simulink library "starslibMathOperations"  (R2024b)
settings: Solver=ode45  StartTime=0.0  StopTime=10.0  RelTol=1e-3  EnableMultiTasking=on
libraries: $bdroot x8
(part 1 of 2)
settings Model: Creator=eheim  LastModifiedBy=gryph
settings SolverCC: AlgebraicLoopSolver=TrustRegion
settings DataIOCC: LimitDataPoints=on  SaveFormat=Array  SignalLoggingSaveFormat=ModelDataLogs  ReturnWorkspaceOutputs=off
settings OptimizationCC: ReuseModelBlockBuffer=off  ExpressionDepthLimit=2147483647  LifeSpan=inf
settings DebuggingCC: UnderspecifiedInitializationDetection=Classic  MergeDetectMultiDrivingBlocksExec=none  SolverPrmCheckMsg=warning  FcnCallInpInsideContextMsg=warning  UnconnectedInputMsg=warning  UnconnectedOutputMsg=warning  UnconnectedLineMsg=warning  StateNameClashWarn=warning  SFUnexpectedBacktrackingDiag=warning  SFNoUnconditionalDefaultTransitionDiag=warning  SFExecutionAtInitializationDiag=none  ArithmeticOperatorsInVariantConditions=warning
settings HardwareCC: ProdBitPerPointer=32  ProdBitPerSizeT=32  ProdBitPerPtrDiffT=32  ProdLargestAtomicFloat=None  ProdIntDivRoundTo=Undefined  ProdEndianess=Unspecified  ProdWordSize=32  ProdHWDeviceType=32-bit Generic
settings ModelReferenceCC: PropagateSignalLabelsOutOfModel=off
settings SFSimCC: SimUseLocalCustomCode=off  CustomCodeUndefinedFunction=UseInterfaceOnly
settings RTWCC: RTWUseLocalCustomCode=off  GPUComputeCapability=3.5
settings CodeAppCC: StateflowObjectComments=on
settings GRTTargetCC: TargetLangStandard=C89/C90 (ANSI)  CombineOutputUpdateFcns=off  GRTInterface=on
settings ConfigComp: CovMetricSettings=dw  CovSaveCumulativeToWorkspaceVar=on  CovSaveSingleToWorkspaceVar=on  CovExternalEMLEnable=off  CovSFcnEnable=off

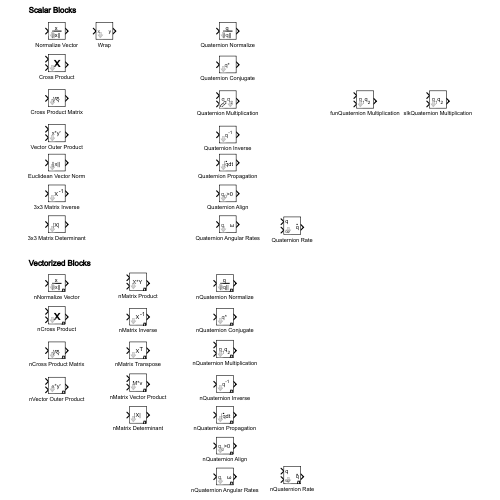
[thumbnail: Simulink's stored preview of the top-level diagram]
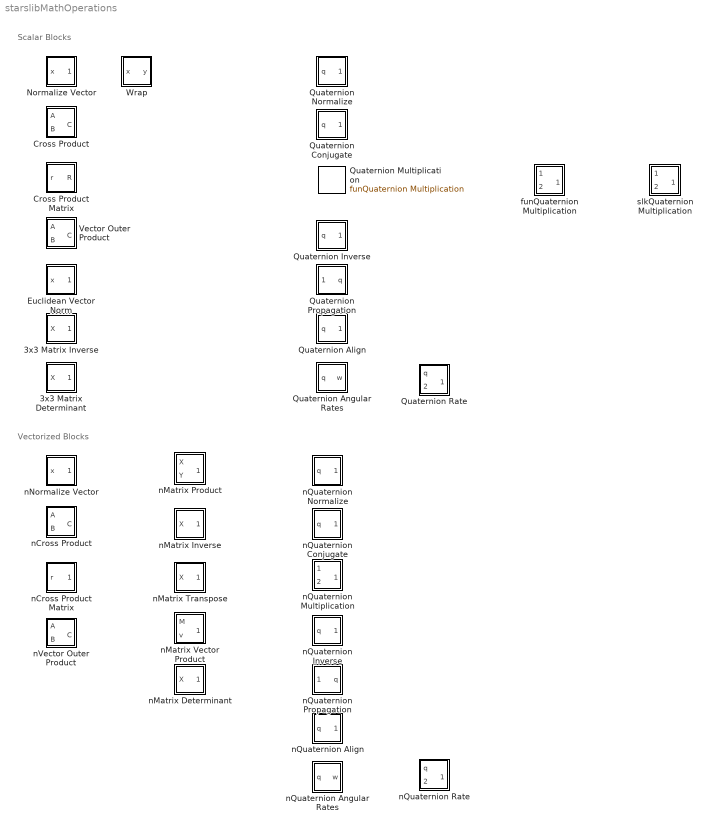
== system starslibMathOperations ==
  note: Scalar Blocks
  note: Vectorized Blocks
  3x3 Matrix Determinant : Subsystem  mask(Matrix Determinant (3x3)){}
      mask help: Determinant of a 3x3 matrix.
      mask Display: text(0.5,0.5,'|X|','HorizontalAlignment','Center','VerticalAlignment','Middle')
  3x3 Matrix Inverse : Subsystem  mask(Matrix Inverse (3x3)){}
      mask help: Inverse of a 3x3 matrix.
      mask Display:
      | text(0.5,0.5,'X','HorizontalAlignment','Center','VerticalAlignment','Middle')
      | text(0.8,0.7,'-1','HorizontalAlignment','Center','VerticalAlignment','Middle')
  Cross Product : Subsystem  mask(Cross Product (1-D)){}
      mask help:
      | Cross product of two 3 element 1-D vectors.  Same as C = cross(A,B) or
      | C = A x B
      |   = [A(2).*B(3) - A(3).*B(2);
      |       A(3).*B(1) - A(1).*B(3);
      |       A(1).*B(2) - A(2).*B(1)];
      mask Display:
      | % plot([0.3 0.7],[0.7 0.3]);
      | % plot([0.3 0.7],[0.3 0.7]);
      |  text(0.575,0.5,'{\fontsize{16}\bfX}','texmode','on','HorizontalAlignment','center',...
      | 	'VerticalAlignment','middle')
  Cross Product Matrix : Subsystem  mask(Cross Product Matrix){n=0}
      mask prompts: n "Hidden variable"
      mask help: Cross product matrix.
      mask Display: text(0.5,0.5,'\{{\itR}\}','texmode', 'on','HorizontalAlignment','Center','VerticalAlignment','Middle')
  Euclidean Vector Norm : Subsystem  mask(Euclidean Norm){dim=1}
      mask prompts: dim "Dimension to take norm"
      mask help: Norm of n-dimensional vector.
      mask Display: text(0.5,0.5,'||x||','texmode', 'on','HorizontalAlignment','Center','VerticalAlignment','Middle')
  Normalize Vector : Subsystem  mask(Normalize Vector){dimnorm=rows, n=1}
      mask prompts: dimnorm "Hidden dimension"; n "Hidden variable"
      mask help: Normalization of 1-dimensional vector.
      mask TypeOptions dimnorm: rows | columns
      mask Display:
      | text(0.5,0.7,'x','HorizontalAlignment','Center','VerticalAlignment','Middle')
      | text(0.5,0.3,'||x||','HorizontalAlignment','Center','VerticalAlignment','Middle')
      | plot([0.2 0.8],[0.5 0.5])
  Quaternion Align : Subsystem  mask(Quaternion Short Path (1-D)){n=0}
      mask prompts: n "Hidden variable"
      mask help: Ensure quaternion transformation takes the shortest possible path. If scalar part is negative the entire quaternion is negated.
      mask Display: text(0.5,0.5,'q_0>0','texmode', 'on','HorizontalAlignment','Center','VerticalAlignment','Middle')
  Quaternion Angular Rates : Subsystem  mask(Quaternion Angular Rates){}
      mask help: Numerically differentiates quaternion and outputs approximation of angular rates.
      mask Display:
      | port_label('input',1,'q','texmode','on')
      | port_label('output',1,'\omega','texmode','on')
  Quaternion Conjugate : Subsystem  mask(Quaternion Conjugate (1-D)){n=0}
      mask prompts: n "Hidden variable"
      mask help: Conjugate of quaternions.
      mask Display: text(0.5,0.5,'q*','HorizontalAlignment','Center','VerticalAlignment','Middle')
  Quaternion Inverse : Subsystem  mask(Quaternion Inverse (1-D)){n=0}
      mask prompts: n "Hidden variable"
      mask help: Inverse of quaternion.
      mask Display: text(0.6,0.6,'q^{-1}','texmode', 'on','HorizontalAlignment','Center','VerticalAlignment','Middle')
  Quaternion Multiplication : $bdroot/funQuaternion Multiplication  n=0
  Quaternion Normalize : Subsystem  mask(Quaternion Normalize (1-D)){n=0}
      mask prompts: n "Hidden variable"
      mask help: Normalization of quaternion.
      mask Display:
      | text(0.5,0.7,'q','HorizontalAlignment','Center','VerticalAlignment','Middle')
      | text(0.5,0.3,'||q||','HorizontalAlignment','Center','VerticalAlignment','Middle')
      | plot([0.2 0.8],[0.5 0.5])
  Quaternion Propagation : Subsystem  mask(Quaternion Propagation (1-D)){qic=[1;0;0;0], k=0.5}
      mask prompts: qic "Initial Quaternion"; k "Stability gain"
      mask help:
      | Integrates dq/dt to propagate a quaternion with algebraic orthonormality stabilization, where:
      |
      |     {dq/dt} = 1/2{q}*{0; omega} + k*lambda*{q}
      |
      | Input, omega is the angular rate of the rotating frame relative to the reference frame in the rotating system's coordinates.
      |
      | Output is the quaternion from the reference coordinate system to the rotating coordinate system.
      |
      | The stability gain parameter, k should be chosen so that k*dT <= 1, where dT is the integration time step.
      mask Help:
      | NASA TN D-5302
      | Zipfel, P. H., Modeling and Simulation of Aerospace Vehicle Dynamics, 2nd Ed., p372
      mask Display:
      | text(0.6,0.5,'\intqdt','texmode', 'on','HorizontalAlignment','Center','VerticalAlignment','Middle')
      | text(0.45,0.85,'\fontsize{20}.','texmode', 'on','HorizontalAlignment','Center','VerticalAlignment','Middle')
  Quaternion Rate : Subsystem  mask(Quaternion Rate){}
      mask help: Computes the quaternion time rate of change.
      mask Display:
      | port_label('input',1,'q')
      | port_label('input',2,'\omega','texmode','on')
      | port_label('output',1,'q')
      | text(0.85,0.80,'\fontsize{20}.','texmode', 'on','HorizontalAlignment','Center','VerticalAlignment','Middle')
  Vector Outer Product : Subsystem  mask(Outer Product (1-D)){n=0}
      mask prompts: n "Hidden variable"
      mask help: Equivilent matlab x(:)*y(:)'
      mask Display: text(0.5,0.5,'x*y''','HorizontalAlignment','Center','VerticalAlignment','Middle')
  Wrap : Subsystem  mask(Wrap Input){R=2*pi, M=0}
      mask prompts: R "Range of output"; M "Minimum of output"
      mask help: Wraps input to specified range with specified minimum.
  funQuaternion Multiplication : Subsystem  mask(Quaternion Multiplication (1-D)){n=0}
      mask prompts: n "Hidden variable"
      mask help: Quaternion multiplication.
      mask Display: text(0.5,0.5,'q_1q_2','texmode','on','HorizontalAlignment','Center','VerticalAlignment','Middle')
  nCross Product : Subsystem  mask(nCross Product){n=1}
      mask prompts: n "Number of Vectors"
      mask help:
      | Cross product of each respective column for two 3xN matricies.  Same as C = cross(A,B) or
      | C = A x B
      |   = [A(2,:).*B(3,:) - A(3,:).*B(2,:);
      |       A(3,:).*B(1,:) - A(1,:).*B(3,:);
      |       A(1,:).*B(2,:) - A(2,:).*B(1,:)];
      mask Display:
      | % plot([0.3 0.7],[0.7 0.3]);
      | % plot([0.3 0.7],[0.3 0.7]);
      | text(0.575,0.5,'{\fontsize{16}\bfX}','texmode','on','HorizontalAlignment','center','VerticalAlignment','middle')
      | text(1,0,'\bf\it{n}','texmode','on','HorizontalAlignment','Right','VerticalAlignment','base')
  nCross Product Matrix : Subsystem  mask(nCross Product Matrix){n=1}
      mask prompts: n "Number of Vectors"
      mask help: Each column corresponds is the cross product matrix, R reshaped into a vector by columns, i.e. R(:). Inputs must be 3xN in size. Outputs are 9xN in size.
      mask init:
      | A = diag([0 1 -1 -1 0 1 1 -1 0]);
      mask Display:
      | text(0.5,0.5,'\{{\itR}\}','texmode', 'on','HorizontalAlignment','Center','VerticalAlignment','Middle')
      | text(1,0,'\bf\it{n}','texmode','on','HorizontalAlignment','Right','VerticalAlignment','base')
  nMatrix Determinant : Subsystem  mask(nMatrix Determinant){n=1}
      mask prompts: n "Number of Matricies"
      mask help: Determinant of set of matricies.
      mask Display:
      | text(0.5,0.5,'|X|','HorizontalAlignment','Center','VerticalAlignment','Middle')
      | text(1,0,'\bf\it{n}','texmode','on','HorizontalAlignment','Right','VerticalAlignment','base')
  nMatrix Inverse : Subsystem  mask(nMatrix Product){n=1}
      mask prompts: n "Number of Matricies"
      mask help:
      | Output reshape(XY(:,k),3,3)
      | corresponds to the matrix product
      | reshape(X(:,k),3,3)*reshape(Y(:,k),3,3)
      |
      | Note: This block has no divide by zero protection.
      mask Display:
      | text(0.5,0.5,'X','HorizontalAlignment','Center','VerticalAlignment','Middle')
      | text(0.8,0.7,'-1','HorizontalAlignment','Center','VerticalAlignment','Middle')
      | text(1,0,'\bf\it{n}','texmode','on','HorizontalAlignment','Right','VerticalAlignment','base')
  nMatrix Product : Subsystem  mask(nMatrix Product){n=1}
      mask prompts: n "Number of Matricies"
      mask help:
      | Output reshape(XY(:,k),3,3)
      | corresponds to the matrix product
      | reshape(X(:,k),3,3)*reshape(Y(:,k),3,3)
      mask Display:
      | text(0.5,0.5,'X*Y','HorizontalAlignment','Center','VerticalAlignment','Middle')
      | text(1,0,'\bf\it{n}','texmode','on','HorizontalAlignment','Right','VerticalAlignment','base')
  nMatrix Transpose : Subsystem  mask(nMatrix Transpose){n=1}
      mask prompts: n "Number of Matricies"
      mask help:
      | Output reshape(AT(:,k),3,3) corresponds
      | to the transpose of reshape(A(:,k),3,3).
      mask Display:
      | text(0.5,0.5,'X','HorizontalAlignment','Center','VerticalAlignment','Middle')
      | text(0.75,0.65,'T','HorizontalAlignment','Center','VerticalAlignment','Middle')
      | text(1,0,'\bf\it{n}','texmode','on','HorizontalAlignment','Right','VerticalAlignment','base')
  nMatrix Vector Product : Subsystem  mask(nMatrix Vector Product){n=1}
      mask prompts: n "Number of Matricies"
      mask help:
      | Output AV(:,k) corresponds to
      | the matrix-vector product
      | reshape(A(:,k),3,3)*V(:,k)
      mask Display:
      | text(0.5,0.5,'M*v','HorizontalAlignment','Center','VerticalAlignment','Middle')
      | text(1,0,'\bf\it{n}','texmode','on','HorizontalAlignment','Right','VerticalAlignment','base')
  nNormalize Vector : Subsystem  mask(nNormalize Vector){dimnorm=rows, n=[3, 1]}
      mask prompts: dimnorm "Dimension to normalize"; n "Dimensions of input [m n]"
      mask help: Normalization of either rows or columns of a 2-dimensional matrix.
      mask init:
      | % Repleat magnitude array, M by A*M*B
      | switch dimnorm
      |     case 1
      |         A = ones(n(1),1);
      |         B = eye(n(2));
      |     case 2
      |         A = eye(n(1));
      |         B  = ones(1,n(2));
      | end
      mask TypeOptions dimnorm: rows | columns
      mask Display:
      | text(0.5,0.7,'x','HorizontalAlignment','Center','VerticalAlignment','Middle')
      | text(0.5,0.3,'||x||','HorizontalAlignment','Center','VerticalAlignment','Middle')
      | plot([0.2 0.8],[0.5 0.5])
      | text(1,0,'\bf\it{n}','texmode','on','HorizontalAlignment','Right','VerticalAlignment','base')
  nQuaternion Align : Subsystem  mask(nQuaternion Align){n=1}
      mask prompts: n "Number of Quaternions"
      mask help: Ensure quaternion transformation takes the shortest possible path. If scalar part is negative the entire quaternion is negated.
      mask Display:
      | text(0.5,0.5,'q_0>0','texmode', 'on','HorizontalAlignment','Center','VerticalAlignment','Middle')
      | text(1,0,'\bf\it{n}','texmode','on','HorizontalAlignment','Right','VerticalAlignment','base')
  nQuaternion Angular Rates : Subsystem  mask(nQuaternion Angular Rates){n=0}
      mask prompts: n "Number of Quaternions"
      mask help: Numerically differentiates quaternion and outputs approximation of angular rates.
      mask Display:
      | text(1,0,'\bf\it{n}','texmode','on','HorizontalAlignment','Right','VerticalAlignment','base')
      | port_label('input',1,'q','texmode','on')
      | port_label('output',1,'\omega','texmode','on')
  nQuaternion Conjugate : Subsystem  mask(nQuaternion Conjugate){n=1}
      mask prompts: n "Number of Quaternions"
      mask help: Conjugate of quaternions.
      mask Display:
      | text(0.5,0.5,'q*','HorizontalAlignment','Center','VerticalAlignment','Middle')
      | text(1,0,'\bf\it{n}','texmode','on','HorizontalAlignment','Right','VerticalAlignment','base')
  nQuaternion Inverse : Subsystem  mask(nQuaternion Inverse){n=1}
      mask prompts: n "Number of Quaternions"
      mask help: Inverse of quaternions.
      mask Display:
      | text(0.6,0.6,'q^{-1}','texmode', 'on','HorizontalAlignment','Center','VerticalAlignment','Middle')
      | text(1,0,'\bf\it{n}','texmode','on','HorizontalAlignment','Right','VerticalAlignment','base')
  nQuaternion Multiplication : Subsystem  mask(nQuaternion Multiplication){n=1}
      mask prompts: n "Number of Quaternions"
      mask help:
      | Quaternion multiplication of two sets of quaternions
      | inputted by 2 (4 x nQuat) matrices
      mask Display:
      | text(0.5,0.5,'q_1q_2','texmode','on','HorizontalAlignment','Center','VerticalAlignment','Middle')
      | text(1,0,'\bf\it{n}','texmode','on','HorizontalAlignment','Right','VerticalAlignment','base')
  nQuaternion Normalize : Subsystem  mask(nQuaternion Normalize){n=1}
      mask prompts: n "Number of Quaternions"
      mask help: Normalization of quaternion.
      mask Display:
      | text(0.5,0.7,'q','HorizontalAlignment','Center','VerticalAlignment','Middle')
      | text(0.5,0.3,'||q||','HorizontalAlignment','Center','VerticalAlignment','Middle')
      | plot([0.2 0.8],[0.5 0.5])
      | text(1,0,'\bf\it{n}','texmode','on','HorizontalAlignment','Right','VerticalAlignment','base')
  nQuaternion Propagation : Subsystem  mask(nQuaternion Propagation){n=1, q0=[1;0;0;0], k=0.5}
      mask prompts: n "Number of Quaternions"; q0 "Initial Quaternion(s)"; k "Stability gain"
      mask help:
      | Integrates dq/dt to propagate a quaternion with algebraic orthonormality stabilization, where:
      |
      |     {dq/dt} = 1/2{q}*{0; omega} + k*lambda*{q}
      |
      | Input, omega is the angular rate of the rotating frame relative to the reference frame in the rotating system's coordinates.
      |
      | Output is the quaternion from the reference coordinate system to the rotating coordinate system.
      |
      | The stability gain parameter, k should be chosen so that k*dT <= 1, where dT is the integration time step.
      mask Help:
      | NASA TN D-5302
      | Zipfel, P. H., Modeling and Simulation of Aerospace Vehicle Dynamics, 2nd Ed., p372
      mask Display:
      | text(0.6,0.5,'\intqdt','texmode', 'on','HorizontalAlignment','Center','VerticalAlignment','Middle')
      | text(0.45,0.85,'\fontsize{20}.','texmode', 'on','HorizontalAlignment','Center','VerticalAlignment','Middle')
      | text(1,0,'\bf\it{n}','texmode','on','HorizontalAlignment','Right','VerticalAlignment','base')
  nQuaternion Rate : Subsystem  mask(Quaternion Rate){n=1}
      mask prompts: n "Number of quaternions in input"
      mask help: Computes the quaternion time rate of change.
      mask Display:
      | port_label('input',1,'q')
      | port_label('input',2,'\omega','texmode','on')
      | port_label('output',1,'q')
      | text(0.85,0.80,'\fontsize{20}.','texmode', 'on','HorizontalAlignment','Center','VerticalAlignment','Middle')
      | text(1,0,'\bf\it{n}','texmode','on','HorizontalAlignment','Right','VerticalAlignment','base')
  nVector Outer Product : Subsystem  mask(nOuter Product){n=1}
      mask prompts: n "Number of Vectors"
      mask help:
      | reshape(OP(:,k),3,3) corresponds
      | to the outer product matrix defined
      | by input X(:,k)*Y(:,k)'.
      mask Display:
      | text(0.5,0.5,'x*y''','HorizontalAlignment','Center','VerticalAlignment','Middle')
      | text(1,0,'\bf\it{n}','texmode','on','HorizontalAlignment','Right','VerticalAlignment','base')
  slkQuaternion Multiplication : Subsystem  mask(Quaternion Multiplication (1-D)){n=0}
      mask prompts: n "Hidden variable"
      mask help: Quaternion multiplication.
      mask Display: text(0.5,0.5,'q_1q_2','texmode','on','HorizontalAlignment','Center','VerticalAlignment','Middle')

== system starslibMathOperations/3x3 Matrix Determinant ==
  X : Inport  PortDimensions=[3,3]
  Reshape : Reshape  OutputDimensionality=Column vector (2-D)
  nMatrix Determinant : $bdroot/nMatrix Determinant  n=1
  inv(X) : Outport  PortDimensions=[1,1]
  wires:
  Reshape/1 -> nMatrix Determinant/1
  X/1 -> Reshape/1
  nMatrix Determinant/1 -> inv(X)/1

== system starslibMathOperations/3x3 Matrix Inverse ==
  X : Inport
  3x3 Matrix Determinant : $bdroot/3x3 Matrix Determinant
  Assertion : Assertion  AssertionFailFcn="disp('Matrix inverse failed.  Matrix is singular.')"
  Product : Product  Inputs=/  Multiplication=Matrix(*)  RndMeth=Zero
  inv(X) : Outport
  wires:
  Product/1 -> inv(X)/1
  X/1 -> Product/1, 3x3 Matrix Determinant/1
  3x3 Matrix Determinant/1 -> Assertion/1

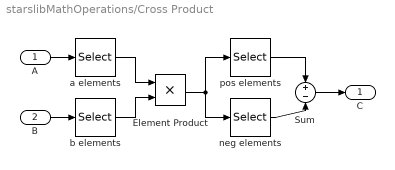
== system starslibMathOperations/Cross Product ==
  A : Inport
  B : Inport  Port=2
  Element Product : Product  RndMeth=Zero
  Sum : Sum  Inputs=+|-
  a elements : Selector  InputPortWidth=3  IndexOptions=Index vector (dialog)  Indices=[2 3 1 3 1 2]  OutputSizes=1
  b elements : Selector  InputPortWidth=3  IndexOptions=Index vector (dialog)  Indices=[3 1 2 2 3 1]  OutputSizes=1
  neg elements : Selector  InputPortWidth=6  IndexOptions=Index vector (dialog)  Indices=[4:6]  OutputSizes=1
  pos elements : Selector  InputPortWidth=6  IndexOptions=Index vector (dialog)  Indices=[1:3]  OutputSizes=1
  C : Outport
  wires:
  a elements/1 -> Element Product/1
  b elements/1 -> Element Product/2
  Element Product/1 -> pos elements/1, neg elements/1
  pos elements/1 -> Sum/1
  neg elements/1 -> Sum/2
  Sum/1 -> C/1
  A/1 -> a elements/1
  B/1 -> b elements/1

== system starslibMathOperations/Cross Product Matrix ==
  r : Inport
  Constant : Constant  Value=[0 1 -1 -1 0 1 1 -1 0]
  Product : Product  RndMeth=Zero
  Reshape : Reshape  OutputDimensionality=Customize  OutputDimensions=[3,3]
  Selector : Selector  InputPortWidth=3  IndexOptions=Index vector (dialog)  Indices=[1 3 2 3 2 1 2 1 3]  OutputSizes=1
  R : Outport  PortDimensions=[3,3]
  wires:
  Reshape/1 -> R/1
  Product/1 -> Reshape/1
  Selector/1 -> Product/2
  r/1 -> Selector/1
  Constant/1 -> Product/1

== system starslibMathOperations/Euclidean Vector Norm ==
  x : Inport
  Math Function : Math  Operator=square  SignedPower=on
  Sqrt : Sqrt
  Sum of Elements : Sum  Inputs=+  CollapseMode=Specified dimension  CollapseDim=dim
  ||x|| : Outport
  wires:
  Sqrt/1 -> ||x||/1
  x/1 -> Math Function/1
  Sum of Elements/1 -> Sqrt/1
  Math Function/1 -> Sum of Elements/1

== system starslibMathOperations/Normalize Vector ==
  x : Inport
  Divide : Product  Inputs=*/
  Math Function : Math  Operator=square  SignedPower=on
  Sqrt : Sqrt
  Sum of Elements : Sum  Inputs=+  CollapseDim=dim
  ux : Outport
  wires:
  Sum of Elements/1 -> Sqrt/1
  Math Function/1 -> Sum of Elements/1
  x/1 -> Math Function/1, Divide/1
  Divide/1 -> ux/1
  Sqrt/1 -> Divide/2

== system starslibMathOperations/Quaternion Align ==
  q : Inport
  Selector2 : Selector  InputPortWidth=4  IndexOptions=Index vector (dialog)  Indices=1  OutputSizes=1
  Switch : Switch  Criteria=u2 > Threshold  ZeroCross=off  SaturateOnIntegerOverflow=off  InputSameDT=off
  Unary Minus : UnaryMinus
  short(q) : Outport
  wires:
  Unary Minus/1 -> Switch/3
  Selector2/1 -> Switch/2
  Switch/1 -> short(q)/1
  q/1 -> Unary Minus/1, Switch/1, Selector2/1

== system starslibMathOperations/Quaternion Angular Rates ==
  q : Inport  PortDimensions=4
  Derivative1 : Derivative
  Gain : Gain  Gain=2
  Gain1 : Gain  Gain=[-1 -1 -1, 1 -1 1, 1 1 -1, -1 1 1]'
  Product3 : Product  Multiplication=Matrix(*)  RndMeth=Zero
  Reshape : Reshape  OutputDimensionality=Customize  OutputDimensions=[3,4]
  Selector3 : Selector  InputPortWidth=4  IndexOptions=Index vector (dialog)  Indices=[2 3 4, 1 4 3, 4 1 2, 3 2 1]  OutputSizes=1
  w : Outport  PortDimensions=3
  wires:
  Selector3/1 -> Gain1/1
  Gain1/1 -> Reshape/1
  Reshape/1 -> Product3/1
  q/1 -> Selector3/1, Derivative1/1
  Product3/1 -> Gain/1
  Gain/1 -> w/1
  Derivative1/1 -> Product3/2

== system starslibMathOperations/Quaternion Conjugate ==
  q : Inport
  Constant : Constant  Value=[1 -1 -1 -1]
  Product : Product  RndMeth=Zero
  q* : Outport
  wires:
  Product/1 -> q*/1
  Constant/1 -> Product/1
  q/1 -> Product/2

== system starslibMathOperations/Quaternion Inverse ==
  q : Inport
  Math Function1 : Math  Operator=square  SignedPower=on
  Product : Product  Inputs=*/  RndMeth=Zero
  Quaternion Conjugate : $bdroot/Quaternion Conjugate  n=0
  Sum of Elements : Sum  Inputs=+
  inv(q) : Outport
  wires:
  Math Function1/1 -> Sum of Elements/1
  Quaternion Conjugate/1 -> Product/1
  q/1 -> Math Function1/1, Quaternion Conjugate/1
  Sum of Elements/1 -> Product/2
  Product/1 -> inv(q)/1

== system starslibMathOperations/Quaternion Normalize ==
  q : Inport
  Math Function1 : Math  Operator=square  SignedPower=on
  Product : Product  Inputs=*/  RndMeth=Zero
  Sqrt : Sqrt
  Sum of Elements : Sum  Inputs=+
  q/||q|| : Outport
  wires:
  Math Function1/1 -> Sum of Elements/1
  Sum of Elements/1 -> Sqrt/1
  Product/1 -> q/||q||/1
  Sqrt/1 -> Product/2
  q/1 -> Math Function1/1, Product/1

== system starslibMathOperations/Quaternion Propagation ==
  Omega : Inport
  Integrator : Integrator  InitialCondition=qic
  Orthonormality Error : Subsystem
      mask Display: text(0.5,0.5,'\lambda','texmode', 'on','HorizontalAlignment','Center','VerticalAlignment','Middle')
  Product : Product  RndMeth=Zero
  Quaternion Rate : $bdroot/Quaternion Rate
  Sum : Sum  Inputs=|++
  k : Gain  Gain=k
  q : Outport
  wires:
  Product/1 -> Sum/2
  k/1 -> Product/1
  Orthonormality Error/1(lambda) -> k/1
  Quaternion Rate/1 -> Sum/1
  Sum/1 -> Integrator/1
  Integrator/1 -> Product/2, Quaternion Rate/1, Orthonormality Error/1(q), q/1
  Omega/1 -> Quaternion Rate/2

== system starslibMathOperations/Quaternion Rate ==
  q : Inport
  Omega : Inport  Port=2
  Gain : Gain  Gain=0.5
  Subsystem6 : Subsystem  mask(Quat Mult for two special sets of quaternions){}
      mask help:
      | Quaternion multiplication of two sets of quaternions. First element assumed
      | zero of second Quaternion.  Input only last three elements
      | of second quaternion.
      mask Display:
      | disp('Quat Mult\n q0=0')
      | port_label('input',1,'p')
      | port_label('input',2,'q')
      | port_label('output',1,'p*q')
  qdt : Outport
  wires:
  Omega/1 -> Subsystem6/2(q)
  Gain/1 -> qdt/1
  q/1 -> Subsystem6/1(p)
  Subsystem6/1(p * q) -> Gain/1

== system starslibMathOperations/Vector Outer Product ==
  A : Inport
  B : Inport  Port=2
  Element Product : Product  RndMeth=Zero
  Reshape : Reshape  OutputDimensionality=Customize  OutputDimensions=[3,3]
  a elements : Selector  InputPortWidth=3  IndexOptions=Index vector (dialog)  Indices=[1 2 3 1 2 3 1 2 3]  OutputSizes=1
  b elements : Selector  InputPortWidth=3  IndexOptions=Index vector (dialog)  Indices=[1 1 1 2 2 2 3 3 3]  OutputSizes=1
  C : Outport
  wires:
  Reshape/1 -> C/1
  a elements/1 -> Element Product/1
  b elements/1 -> Element Product/2
  A/1 -> a elements/1
  B/1 -> b elements/1
  Element Product/1 -> Reshape/1

== system starslibMathOperations/Wrap ==
  x : Inport
  Min : Constant  Value=M  VectorParams1D=off
  Range : Constant  Value=R  VectorParams1D=off
  Sum : Sum  Inputs=|+-
  Sum1 : Sum  Inputs=|++
  mod : Math  Operator=mod  SignedPower=on
  y : Outport
  wires:
  Sum1/1 -> y/1
  x/1 -> Sum/1
  Sum/1 -> mod/1
  Range/1 -> mod/2
  mod/1 -> Sum1/1
  Min/1 -> Sum1/2, Sum/2

== system starslibMathOperations/funQuaternion Multiplication ==
  q1 : Inport
  q2 : Inport  Port=2
  Quaternion Multiplication : MATLAB Function  TreatAsAtomicUnit=on
  q1q2 : Outport
  wires:
  Quaternion Multiplication/1(q1q2) -> q1q2/1
  q2/1 -> Quaternion Multiplication/2(q2)
  q1/1 -> Quaternion Multiplication/1(q1)

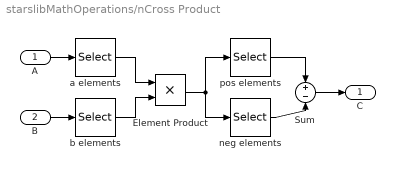
== system starslibMathOperations/nCross Product ==
  A : Inport  PortDimensions=[3,n]
  B : Inport  Port=2  PortDimensions=[3,n]
  Element Product : Product  RndMeth=Zero
  Sum : Sum  Inputs=+|-
  a elements : Selector  NumberOfDimensions=2  InputPortWidth=3  IndexOptions=Index vector (dialog),Select all  Indices=[2 3 1 3 1 2],1  OutputSizes=1,1
  b elements : Selector  NumberOfDimensions=2  InputPortWidth=3  IndexOptions=Index vector (dialog),Select all  Indices=[3 1 2 2 3 1],1  OutputSizes=1,1
  neg elements : Selector  NumberOfDimensions=2  InputPortWidth=3  IndexOptions=Index vector (dialog),Select all  Indices=[4:6],1  OutputSizes=1,1
  pos elements : Selector  NumberOfDimensions=2  InputPortWidth=3  IndexOptions=Index vector (dialog),Select all  Indices=[1:3],1  OutputSizes=1,1
  C : Outport  PortDimensions=[3,n]
  wires:
  a elements/1 -> Element Product/1
  b elements/1 -> Element Product/2
  Element Product/1 -> pos elements/1, neg elements/1
  pos elements/1 -> Sum/1
  neg elements/1 -> Sum/2
  Sum/1 -> C/1
  A/1 -> a elements/1
  B/1 -> b elements/1

== system starslibMathOperations/nCross Product Matrix ==
  r : Inport  PortDimensions=[3,n]
  Constant : Constant  Value=A
  Product : Product  Multiplication=Matrix(*)  RndMeth=Zero
  Selector : Selector  NumberOfDimensions=2  InputPortWidth=3  IndexOptions=Index vector (dialog),Select all  Indices=[1 3 2 3 2 1 2 1 3],1  OutputSizes=1,1
  nR(:) : Outport  PortDimensions=[9,n]
  wires:
  Product/1 -> nR(:)/1
  Selector/1 -> Product/2
  r/1 -> Selector/1
  Constant/1 -> Product/1

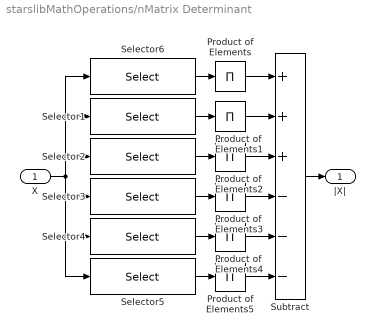
== system starslibMathOperations/nMatrix Determinant ==
  X : Inport  PortDimensions=[9,n]
  Product of Elements{,1..5} (6 alike) : Product  Inputs=*  CollapseMode=Specified dimension
  Selector1 : Selector  NumberOfDimensions=2  InputPortWidth=3  IndexOptions=Index vector (dialog),Select all  Indices=[4 8 3],1  OutputSizes=1,1
  Selector2 : Selector  NumberOfDimensions=2  InputPortWidth=3  IndexOptions=Index vector (dialog),Select all  Indices=[7 2 6],1  OutputSizes=1,1
  Selector3 : Selector  NumberOfDimensions=2  InputPortWidth=3  IndexOptions=Index vector (dialog),Select all  Indices=[7 5 3],1  OutputSizes=1,1
  Selector4 : Selector  NumberOfDimensions=2  InputPortWidth=3  IndexOptions=Index vector (dialog),Select all  Indices=[4 2 9],1  OutputSizes=1,1
  Selector5 : Selector  NumberOfDimensions=2  InputPortWidth=3  IndexOptions=Index vector (dialog),Select all  Indices=[1 8 6],1  OutputSizes=1,1
  Selector6 : Selector  NumberOfDimensions=2  InputPortWidth=3  IndexOptions=Index vector (dialog),Select all  Indices=[1 5 9],1  OutputSizes=1,1
  Subtract : Sum  Inputs=+++---
  |X| : Outport  PortDimensions=[1,n]
  wires:
  Selector6/1 -> Product of Elements/1
  Selector1/1 -> Product of Elements1/1
  Selector2/1 -> Product of Elements2/1
  Selector3/1 -> Product of Elements3/1
  Selector4/1 -> Product of Elements4/1
  Selector5/1 -> Product of Elements5/1
  X/1 -> Selector2/1, Selector6/1, Selector1/1, Selector3/1, Selector5/1, Selector4/1
  Product of Elements/1 -> Subtract/1
  Product of Elements1/1 -> Subtract/2
  Product of Elements2/1 -> Subtract/3
  Product of Elements3/1 -> Subtract/4
  Product of Elements4/1 -> Subtract/5
  Product of Elements5/1 -> Subtract/6
  Subtract/1 -> |X|/1

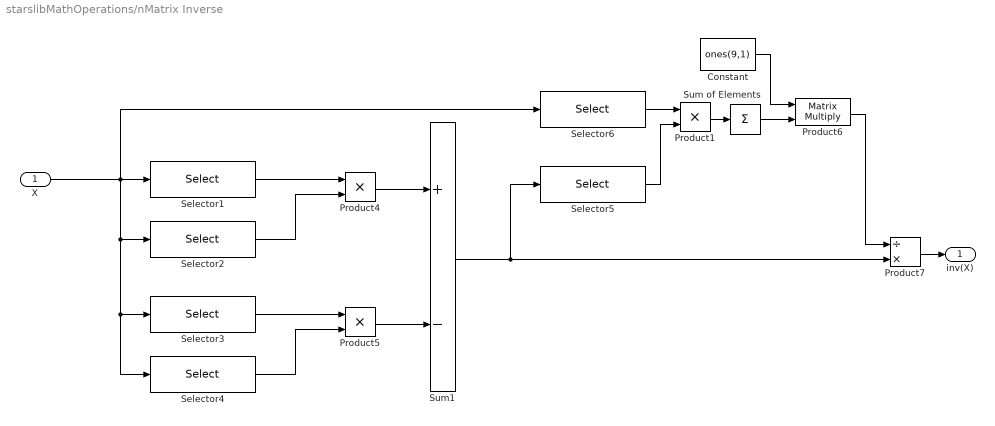
== system starslibMathOperations/nMatrix Inverse ==
  X : Inport  PortDimensions=[9,n]
  Constant : Constant  Value=ones(9,1)  VectorParams1D=off
  Product1 : Product  RndMeth=Zero
  Product4 : Product  RndMeth=Zero
  Product5 : Product  RndMeth=Zero
  Product6 : Product  Multiplication=Matrix(*)  RndMeth=Zero
  Product7 : Product  Inputs=/*  RndMeth=Zero
  Selector1 : Selector  NumberOfDimensions=2  InputPortWidth=3  IndexOptions=Index vector (dialog),Select all  Indices=[5 8 2 7 1 4 4 7 1],1  OutputSizes=1,1
  Selector2 : Selector  NumberOfDimensions=2  InputPortWidth=3  IndexOptions=Index vector (dialog),Select all  Indices=[9 3 6 6 9 3 8 2 5],1  OutputSizes=1,1
  Selector3 : Selector  NumberOfDimensions=2  InputPortWidth=3  IndexOptions=Index vector (dialog),Select all  Indices=[8 2 5 4 7 1 7 1 4],1  OutputSizes=1,1
  Selector4 : Selector  NumberOfDimensions=2  InputPortWidth=3  IndexOptions=Index vector (dialog),Select all  Indices=[6 9 3 9 3 6 5 8 2],1  OutputSizes=1,1
  Selector5 : Selector  NumberOfDimensions=2  InputPortWidth=3  IndexOptions=Index vector (dialog),Select all  Indices=[1 2 3],1  OutputSizes=1,1
  Selector6 : Selector  NumberOfDimensions=2  InputPortWidth=3  IndexOptions=Index vector (dialog),Select all  Indices=[1 4 7],1  OutputSizes=1,1
  Sum of Elements : Sum  Inputs=+  CollapseMode=Specified dimension
  Sum1 : Sum  Inputs=+-
  inv(X) : Outport  PortDimensions=[9,n]
  wires:
  Product7/1 -> inv(X)/1
  Product6/1 -> Product7/1
  Constant/1 -> Product6/1
  Sum of Elements/1 -> Product6/2
  Product1/1 -> Sum of Elements/1
  Selector5/1 -> Product1/2
  Selector6/1 -> Product1/1
  Sum1/1 -> Product7/2, Selector5/1
  Product5/1 -> Sum1/2
  Product4/1 -> Sum1/1
  Selector4/1 -> Product5/2
  Selector3/1 -> Product5/1
  Selector2/1 -> Product4/2
  Selector1/1 -> Product4/1
  X/1 -> Selector6/1, Selector2/1, Selector4/1, Selector3/1, Selector1/1

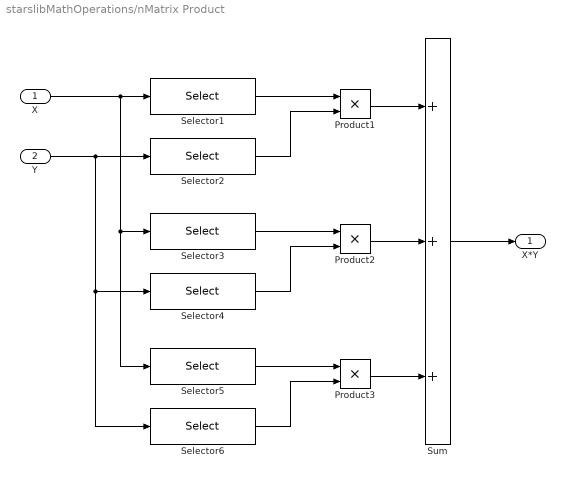
== system starslibMathOperations/nMatrix Product ==
  X : Inport  PortDimensions=[9,n]
  Y : Inport  Port=2  PortDimensions=[9,n]
  Product1 : Product  RndMeth=Zero
  Product2 : Product  RndMeth=Zero
  Product3 : Product  RndMeth=Zero
  Selector1 : Selector  NumberOfDimensions=2  InputPortWidth=3  IndexOptions=Index vector (dialog),Select all  Indices=[1 2 3 1 2 3 1 2 3],1  OutputSizes=1,1
  Selector2 : Selector  NumberOfDimensions=2  InputPortWidth=3  IndexOptions=Index vector (dialog),Select all  Indices=[1 1 1 4 4 4 7 7 7],1  OutputSizes=1,1
  Selector3 : Selector  NumberOfDimensions=2  InputPortWidth=3  IndexOptions=Index vector (dialog),Select all  Indices=[4 5 6 4 5 6 4 5 6],1  OutputSizes=1,1
  Selector4 : Selector  NumberOfDimensions=2  InputPortWidth=3  IndexOptions=Index vector (dialog),Select all  Indices=[2 2 2 5 5 5 8 8 8],1  OutputSizes=1,1
  Selector5 : Selector  NumberOfDimensions=2  InputPortWidth=3  IndexOptions=Index vector (dialog),Select all  Indices="[7 8 9  7 8 9 7 8 9],1"  OutputSizes=1,1
  Selector6 : Selector  NumberOfDimensions=2  InputPortWidth=3  IndexOptions=Index vector (dialog),Select all  Indices=[3 3 3 6 6 6 9 9 9],1  OutputSizes=1,1
  Sum : Sum  Inputs=+++
  X*Y : Outport  PortDimensions=[9,n]
  wires:
  Sum/1 -> X*Y/1
  Product3/1 -> Sum/3
  Product2/1 -> Sum/2
  Product1/1 -> Sum/1
  Selector6/1 -> Product3/2
  Selector5/1 -> Product3/1
  Selector4/1 -> Product2/2
  Selector3/1 -> Product2/1
  Selector2/1 -> Product1/2
  Selector1/1 -> Product1/1
  Y/1 -> Selector2/1, Selector4/1, Selector6/1
  X/1 -> Selector1/1, Selector3/1, Selector5/1

== system starslibMathOperations/nMatrix Transpose ==
  X : Inport  PortDimensions=[9,n]
  Selector1 : Selector  NumberOfDimensions=2  InputPortWidth=3  IndexOptions=Index vector (dialog),Select all  Indices=[1 4 7 2 5 8 3 6 9],1  OutputSizes=1,1
  X^T : Outport  PortDimensions=[9,n]
  wires:
  Selector1/1 -> X^T/1
  X/1 -> Selector1/1

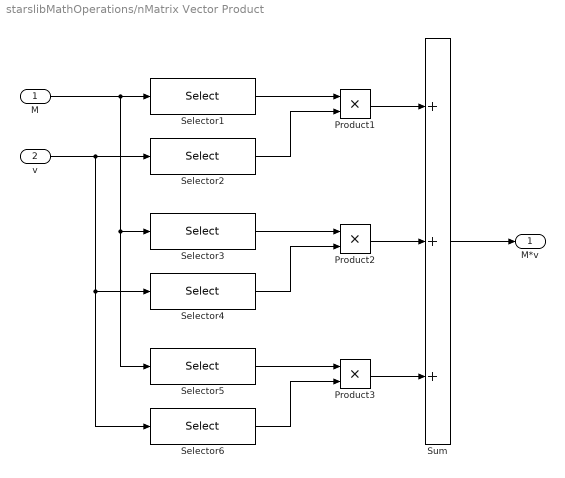
== system starslibMathOperations/nMatrix Vector Product ==
  M : Inport  PortDimensions=[9,n]
  v : Inport  Port=2  PortDimensions=[3,n]
  Product1 : Product  RndMeth=Zero
  Product2 : Product  RndMeth=Zero
  Product3 : Product  RndMeth=Zero
  Selector1 : Selector  NumberOfDimensions=2  InputPortWidth=3  IndexOptions=Index vector (dialog),Select all  Indices=[1 2 3],1  OutputSizes=1,1
  Selector2 : Selector  NumberOfDimensions=2  InputPortWidth=3  IndexOptions=Index vector (dialog),Select all  Indices=[1 1 1],1  OutputSizes=1,1
  Selector3 : Selector  NumberOfDimensions=2  InputPortWidth=3  IndexOptions=Index vector (dialog),Select all  Indices=[4 5 6],1  OutputSizes=1,1
  Selector4 : Selector  NumberOfDimensions=2  InputPortWidth=3  IndexOptions=Index vector (dialog),Select all  Indices=[2 2 2],1  OutputSizes=1,1
  Selector5 : Selector  NumberOfDimensions=2  InputPortWidth=3  IndexOptions=Index vector (dialog),Select all  Indices=[7 8 9],1  OutputSizes=1,1
  Selector6 : Selector  NumberOfDimensions=2  InputPortWidth=3  IndexOptions=Index vector (dialog),Select all  Indices=[3 3 3],1  OutputSizes=1,1
  Sum : Sum  Inputs=+++
  M*v : Outport  PortDimensions=[3,n]
  wires:
  Sum/1 -> M*v/1
  Product3/1 -> Sum/3
  Product2/1 -> Sum/2
  Product1/1 -> Sum/1
  Selector6/1 -> Product3/2
  Selector5/1 -> Product3/1
  Selector4/1 -> Product2/2
  Selector3/1 -> Product2/1
  Selector2/1 -> Product1/2
  Selector1/1 -> Product1/1
  v/1 -> Selector2/1, Selector4/1, Selector6/1
  M/1 -> Selector1/1, Selector3/1, Selector5/1

== system starslibMathOperations/nNormalize Vector ==
  x : Inport  PortDimensions=n
  Divide : Product  Inputs=*/
  Divide by Zero Protection : Subsystem
  Euclidean Vector Norm : $bdroot/Euclidean Vector Norm  dim=1
  Repeat Diminsion : Subsystem
  ux : Outport  PortDimensions=n
  wires:
  Repeat Diminsion/1(Rep M*) -> Divide/2
  x/1 -> Divide/1, Euclidean Vector Norm/1
  Divide by Zero Protection/1(M*) -> Repeat Diminsion/1(M*)
  Divide/1 -> ux/1
  Euclidean Vector Norm/1 -> Divide by Zero Protection/1(M)

== system starslibMathOperations/nQuaternion Align ==
  q : Inport  PortDimensions=[4,n]
  Selector2 : Selector  NumberOfDimensions=2  InputPortWidth=3  IndexOptions=Index vector (dialog),Select all  Indices=1,1  OutputSizes=1,1
  Switch : Switch  Criteria=u2 > Threshold  ZeroCross=off  SaturateOnIntegerOverflow=off  InputSameDT=off
  Unary Minus : UnaryMinus
  short(q) : Outport  PortDimensions=[4,n]
  wires:
  Unary Minus/1 -> Switch/3
  Selector2/1 -> Switch/2
  Switch/1 -> short(q)/1
  q/1 -> Unary Minus/1, Selector2/1, Switch/1

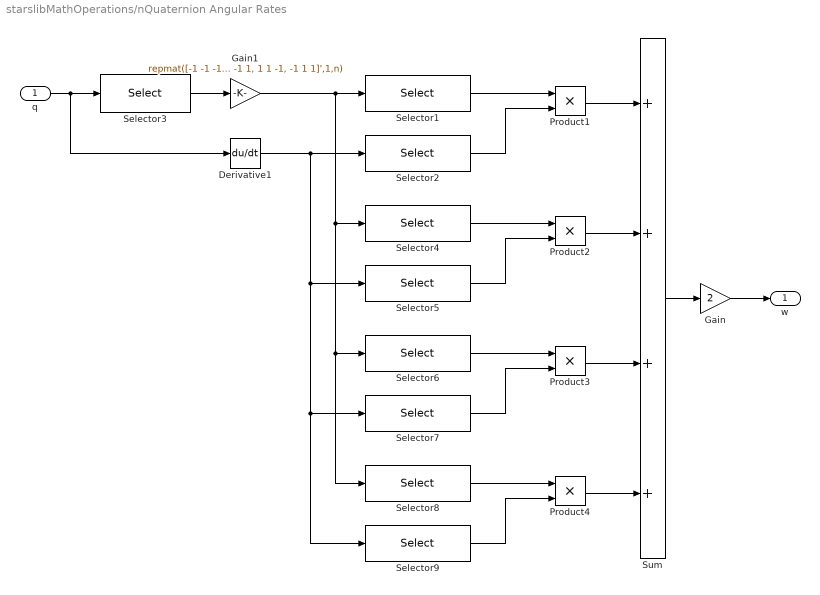
== system starslibMathOperations/nQuaternion Angular Rates ==
  q : Inport  PortDimensions=[4,n]
  Derivative1 : Derivative
  Gain : Gain  Gain=2
  Gain1 : Gain  Gain=repmat([-1 -1 -1, 1 -1 1, 1 1 -1, -1 1 1]',1,n)
  Product{1..4} (4 alike) : Product  RndMeth=Zero
  Selector1 : Selector  NumberOfDimensions=2  InputPortWidth=3  IndexOptions=Index vector (dialog),Select all  Indices=[1 2 3],1  OutputSizes=1,1
  Selector2 : Selector  NumberOfDimensions=2  InputPortWidth=3  IndexOptions=Index vector (dialog),Select all  Indices=[1 1 1],1  OutputSizes=1,1
  Selector3 : Selector  NumberOfDimensions=2  InputPortWidth=4  IndexOptions=Index vector (dialog),Select all  Indices=[2 3 4, 1 4 3, 4 1 2, 3 2 1],1  OutputSizes=1,1
  Selector4 : Selector  NumberOfDimensions=2  InputPortWidth=3  IndexOptions=Index vector (dialog),Select all  Indices=[4 5 6],1  OutputSizes=1,1
  Selector5 : Selector  NumberOfDimensions=2  InputPortWidth=3  IndexOptions=Index vector (dialog),Select all  Indices=[2 2 2],1  OutputSizes=1,1
  Selector6 : Selector  NumberOfDimensions=2  InputPortWidth=3  IndexOptions=Index vector (dialog),Select all  Indices=[7 8 9],1  OutputSizes=1,1
  Selector7 : Selector  NumberOfDimensions=2  InputPortWidth=3  IndexOptions=Index vector (dialog),Select all  Indices=[3 3 3],1  OutputSizes=1,1
  Selector8 : Selector  NumberOfDimensions=2  InputPortWidth=3  IndexOptions=Index vector (dialog),Select all  Indices=[10 11 12],1  OutputSizes=1,1
  Selector9 : Selector  NumberOfDimensions=2  InputPortWidth=3  IndexOptions=Index vector (dialog),Select all  Indices=[4 4 4],1  OutputSizes=1,1
  Sum : Sum  Inputs=++++
  w : Outport  PortDimensions=[3,n]
  wires:
  Product4/1 -> Sum/4
  Selector9/1 -> Product4/2
  Selector8/1 -> Product4/1
  Sum/1 -> Gain/1
  Product3/1 -> Sum/3
  Product2/1 -> Sum/2
  Product1/1 -> Sum/1
  Selector7/1 -> Product3/2
  Selector6/1 -> Product3/1
  Selector5/1 -> Product2/2
  Selector4/1 -> Product2/1
  Selector2/1 -> Product1/2
  Selector1/1 -> Product1/1
  Derivative1/1 -> Selector9/1, Selector7/1, Selector5/1, Selector2/1
  Gain1/1 -> Selector8/1, Selector6/1, Selector4/1, Selector1/1
  Gain/1 -> w/1
  q/1 -> Selector3/1, Derivative1/1
  Selector3/1 -> Gain1/1

== system starslibMathOperations/nQuaternion Conjugate ==
  q : Inport  PortDimensions=[4,n]
  Constant3 : Constant  Value=diag([1 -1 -1 -1])  VectorParams1D=off
  Product : Product  Multiplication=Matrix(*)  RndMeth=Zero
  inv(q) : Outport  PortDimensions=[4,n]
  wires:
  Constant3/1 -> Product/1
  q/1 -> Product/2
  Product/1 -> inv(q)/1

== system starslibMathOperations/nQuaternion Inverse ==
  q : Inport  PortDimensions=[4,n]
  Constant : Constant  Value=[1; 1; 1; 1;]  VectorParams1D=off
  Math Function1 : Math  Operator=square  SignedPower=on
  Product : Product  Inputs=*/  RndMeth=Zero
  Product1 : Product  Multiplication=Matrix(*)  RndMeth=Zero
  Sum of Elements : Sum  Inputs=+  CollapseMode=Specified dimension
  nQuaternion Conjugate : $bdroot/nQuaternion Conjugate  n=n
  inv(q) : Outport  PortDimensions=[4,n]
  wires:
  Math Function1/1 -> Sum of Elements/1
  nQuaternion Conjugate/1 -> Product/1
  q/1 -> Math Function1/1, nQuaternion Conjugate/1
  Sum of Elements/1 -> Product1/2
  Constant/1 -> Product1/1
  Product1/1 -> Product/2
  Product/1 -> inv(q)/1

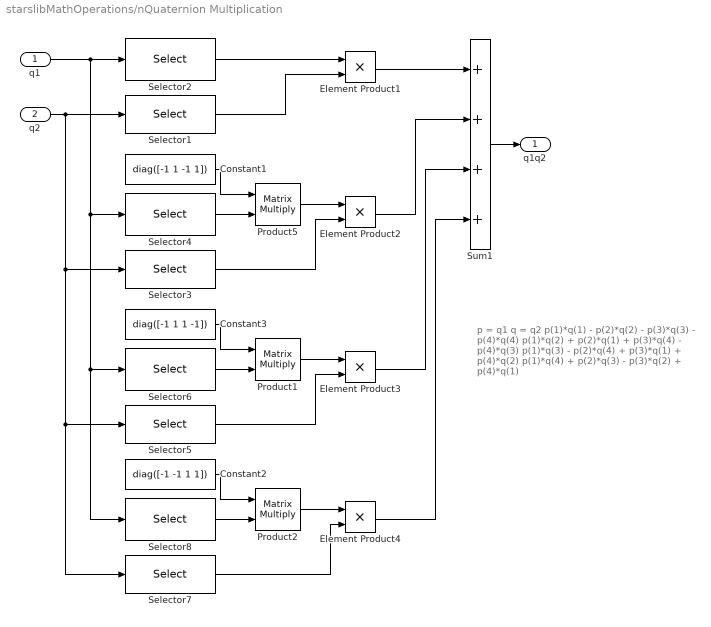
== system starslibMathOperations/nQuaternion Multiplication ==
  note: p = q1
      | q = q2
      |
      | p(1)*q(1) - p(2)*q(2) - p(3)*q(3) - p(4)*q(4)
      |
      | p(1)*q(2) + p(2)*q(1) + p(3)*q(4) - p(4)*q(3)
      |
      | p(1)*q(3) - p(2)*q(4) + p(3)*q(1) + p(4)*q(2)
      |
      | p(1)*q(4) + p(2)*q(3) - p(3)*q(2) + p(4)*q(1)
  q1 : Inport  PortDimensions=[4,n]
  q2 : Inport  Port=2  PortDimensions=[4,n]
  Constant1 : Constant  Value=diag([-1 1 -1 1])  VectorParams1D=off
  Constant2 : Constant  Value=diag([-1 -1 1 1])  VectorParams1D=off
  Constant3 : Constant  Value=diag([-1 1 1 -1])  VectorParams1D=off
  Element Product{1..4} (4 alike) : Product  RndMeth=Zero
  Product1 : Product  Multiplication=Matrix(*)  RndMeth=Zero
  Product2 : Product  Multiplication=Matrix(*)  RndMeth=Zero
  Product5 : Product  Multiplication=Matrix(*)  RndMeth=Zero
  Selector1 : Selector  NumberOfDimensions=2  InputPortWidth=3  IndexOptions=Index vector (dialog),Select all  Indices=[1 2 3 4],1  OutputSizes=1,1
  Selector2 : Selector  NumberOfDimensions=2  InputPortWidth=3  IndexOptions=Index vector (dialog),Select all  Indices=[1 1 1 1],1  OutputSizes=1,1
  Selector3 : Selector  NumberOfDimensions=2  InputPortWidth=3  IndexOptions=Index vector (dialog),Select all  Indices=[2 1 4 3],1  OutputSizes=1,1
  Selector4 : Selector  NumberOfDimensions=2  InputPortWidth=3  IndexOptions=Index vector (dialog),Select all  Indices=[2 2 2 2],1  OutputSizes=1,1
  Selector5 : Selector  NumberOfDimensions=2  InputPortWidth=3  IndexOptions=Index vector (dialog),Select all  Indices=[3 4 1 2],1  OutputSizes=1,1
  Selector6 : Selector  NumberOfDimensions=2  InputPortWidth=3  IndexOptions=Index vector (dialog),Select all  Indices=[3 3 3 3],1  OutputSizes=1,1
  Selector7 : Selector  NumberOfDimensions=2  InputPortWidth=3  IndexOptions=Index vector (dialog),Select all  Indices=[4 3 2 1],1  OutputSizes=1,1
  Selector8 : Selector  NumberOfDimensions=2  InputPortWidth=3  IndexOptions=Index vector (dialog),Select all  Indices=[4 4 4 4],1  OutputSizes=1,1
  Sum1 : Sum  Inputs=++++
  q1q2 : Outport  PortDimensions=[4,n]
  wires:
  Sum1/1 -> q1q2/1
  q2/1 -> Selector1/1, Selector3/1, Selector5/1, Selector7/1
  q1/1 -> Selector2/1, Selector4/1, Selector6/1, Selector8/1
  Element Product4/1 -> Sum1/4
  Element Product3/1 -> Sum1/3
  Element Product2/1 -> Sum1/2
  Element Product1/1 -> Sum1/1
  Selector7/1 -> Element Product4/2
  Product2/1 -> Element Product4/1
  Selector5/1 -> Element Product3/2
  Product1/1 -> Element Product3/1
  Selector3/1 -> Element Product2/2
  Product5/1 -> Element Product2/1
  Selector1/1 -> Element Product1/2
  Selector2/1 -> Element Product1/1
  Constant2/1 -> Product2/1
  Selector8/1 -> Product2/2
  Constant3/1 -> Product1/1
  Selector6/1 -> Product1/2
  Constant1/1 -> Product5/1
  Selector4/1 -> Product5/2

== system starslibMathOperations/nQuaternion Normalize ==
  q : Inport  PortDimensions=[4,n]
  Constant : Constant  Value=[1; 1; 1; 1;]  VectorParams1D=off
  Math Function1 : Math  Operator=square  SignedPower=on
  Product : Product  Inputs=*/  RndMeth=Zero
  Product1 : Product  Multiplication=Matrix(*)  RndMeth=Zero
  Sqrt : Sqrt
  Sum of Elements : Sum  Inputs=+  CollapseMode=Specified dimension
  q/||q|| : Outport  PortDimensions=[4,n]
  wires:
  Math Function1/1 -> Sum of Elements/1
  Sum of Elements/1 -> Sqrt/1
  Product/1 -> q/||q||/1
  Product1/1 -> Product/2
  Constant/1 -> Product1/1
  Sqrt/1 -> Product1/2
  q/1 -> Math Function1/1, Product/1

== system starslibMathOperations/nQuaternion Propagation ==
  Omega : Inport  PortDimensions=[3,n]
  Integrator : Integrator  InitialCondition=q0
  Orthonormality Error : Subsystem
      mask Display:
      | text(0.5,0.5,'\lambda','texmode', 'on','HorizontalAlignment','Center','VerticalAlignment','Middle')
      | text(1,0,'\bf\it{n}','texmode','on','HorizontalAlignment','Right','VerticalAlignment','base')
  Product : Product  RndMeth=Zero
  Sum : Sum  Inputs=|++
  k : Gain  Gain=repmat(k,n,1)  Multiplication=Matrix(K*u)
  nQuaternion Rate : $bdroot/nQuaternion Rate  n=n
  q : Outport  PortDimensions=[4,n]
  wires:
  Integrator/1 -> q/1, Orthonormality Error/1(q), nQuaternion Rate/1, Product/2
  Omega/1 -> nQuaternion Rate/2
  Product/1 -> Sum/2
  k/1 -> Product/1
  Orthonormality Error/1(lambda) -> k/1
  nQuaternion Rate/1 -> Sum/1
  Sum/1 -> Integrator/1

== system starslibMathOperations/nQuaternion Rate ==
  q : Inport  PortDimensions=[4,n]
  Omega : Inport  Port=2  PortDimensions=[3,n]
  Gain : Gain  Gain=0.5
  Subsystem6 : Subsystem  mask(Quat Mult for two special sets of quaternions){nQuat=n}
      mask prompts: nQuat "Number of quaternions in input"
      mask help:
      | Quaternion multiplication of two sets of quaternions
      | inputted by 2 (4 x nQuat) matrices. First element assumed
      | zero of second Quaternion.  Input only last three elements
      | of second quaternion.  Used in Qtrans' first quaternion
      | multiplication
      mask Display:
      | disp('n-Quat Mult\n q0=0')
      | port_label('input',1,'p')
      | port_label('input',2,'q')
      | port_label('output',1,'p*q')
  qdt : Outport  PortDimensions=[4,n]
  wires:
  Subsystem6/1(p * q) -> Gain/1
  q/1 -> Subsystem6/1(p)
  Gain/1 -> qdt/1
  Omega/1 -> Subsystem6/2(q)

== system starslibMathOperations/nVector Outer Product ==
  A : Inport  PortDimensions=[3,n]
  B : Inport  Port=2  PortDimensions=[3,n]
  Element Product : Product  RndMeth=Zero
  a elements : Selector  NumberOfDimensions=2  InputPortWidth=3  IndexOptions=Index vector (dialog),Select all  Indices=[1 2 3 1 2 3 1 2 3],1  OutputSizes=1,1
  b elements : Selector  NumberOfDimensions=2  InputPortWidth=3  IndexOptions=Index vector (dialog),Select all  Indices=[1 1 1 2 2 2 3 3 3],1  OutputSizes=1,1
  C : Outport  PortDimensions=[9,n]
  wires:
  a elements/1 -> Element Product/1
  b elements/1 -> Element Product/2
  A/1 -> a elements/1
  B/1 -> b elements/1
  Element Product/1 -> C/1

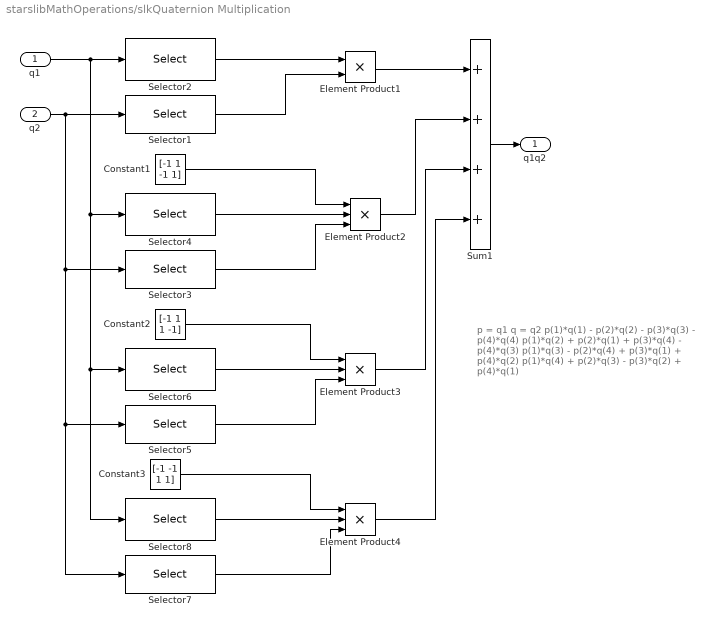
== system starslibMathOperations/slkQuaternion Multiplication ==
  note: p = q1
      | q = q2
      |
      | p(1)*q(1) - p(2)*q(2) - p(3)*q(3) - p(4)*q(4)
      |
      | p(1)*q(2) + p(2)*q(1) + p(3)*q(4) - p(4)*q(3)
      |
      | p(1)*q(3) - p(2)*q(4) + p(3)*q(1) + p(4)*q(2)
      |
      | p(1)*q(4) + p(2)*q(3) - p(3)*q(2) + p(4)*q(1)
  q1 : Inport
  q2 : Inport  Port=2
  Constant1 : Constant  Value=[-1 1 -1 1]
  Constant2 : Constant  Value=[-1 1 1 -1]
  Constant3 : Constant  Value=[-1 -1 1 1]
  Element Product1 : Product  RndMeth=Zero
  Element Product2 : Product  Inputs=3  RndMeth=Zero
  Element Product3 : Product  Inputs=3  RndMeth=Zero
  Element Product4 : Product  Inputs=3  RndMeth=Zero
  Selector1 : Selector  InputPortWidth=4  IndexOptions=Index vector (dialog)  Indices=[1 2 3 4]  OutputSizes=1
  Selector2 : Selector  InputPortWidth=4  IndexOptions=Index vector (dialog)  Indices=[1 1 1 1]  OutputSizes=1
  Selector3 : Selector  InputPortWidth=4  IndexOptions=Index vector (dialog)  Indices=[2 1 4 3]  OutputSizes=1
  Selector4 : Selector  InputPortWidth=4  IndexOptions=Index vector (dialog)  Indices=[2 2 2 2]  OutputSizes=1
  Selector5 : Selector  InputPortWidth=4  IndexOptions=Index vector (dialog)  Indices=[3 4 1 2]  OutputSizes=1
  Selector6 : Selector  InputPortWidth=4  IndexOptions=Index vector (dialog)  Indices=[3 3 3 3]  OutputSizes=1
  Selector7 : Selector  InputPortWidth=4  IndexOptions=Index vector (dialog)  Indices=[4 3 2 1]  OutputSizes=1
  Selector8 : Selector  InputPortWidth=4  IndexOptions=Index vector (dialog)  Indices=[4 4 4 4]  OutputSizes=1
  Sum1 : Sum  Inputs=++++
  q1q2 : Outport
  wires:
  Selector4/1 -> Element Product2/2
  Selector6/1 -> Element Product3/2
  Selector8/1 -> Element Product4/2
  Selector2/1 -> Element Product1/1
  Selector1/1 -> Element Product1/2
  Selector3/1 -> Element Product2/3
  Selector5/1 -> Element Product3/3
  Selector7/1 -> Element Product4/3
  Element Product1/1 -> Sum1/1
  Element Product2/1 -> Sum1/2
  Element Product3/1 -> Sum1/3
  Element Product4/1 -> Sum1/4
  q1/1 -> Selector8/1, Selector6/1, Selector4/1, Selector2/1
  q2/1 -> Selector7/1, Selector5/1, Selector3/1, Selector1/1
  Sum1/1 -> q1q2/1
  Constant1/1 -> Element Product2/1
  Constant2/1 -> Element Product3/1
  Constant3/1 -> Element Product4/1

== system starslibMathOperations/Quaternion Propagation/Orthonormality Error ==
  note: Quaternion orthonormality error.
  note: Zipfel, P. H., Modeling and Simulation of Aerospace Vehicle Dynamics, 2nd Ed., p372
  q : Inport
  Constant : Constant
  Math Function : Math  Operator=square  SignedPower=on
  Sum of Elements : Sum  Inputs=+
  Sum1 : Sum  Inputs=|+-
  lambda : Outport
  wires:
  Sum1/1 -> lambda/1
  q/1 -> Math Function/1
  Sum of Elements/1 -> Sum1/2
  Math Function/1 -> Sum of Elements/1
  Constant/1 -> Sum1/1

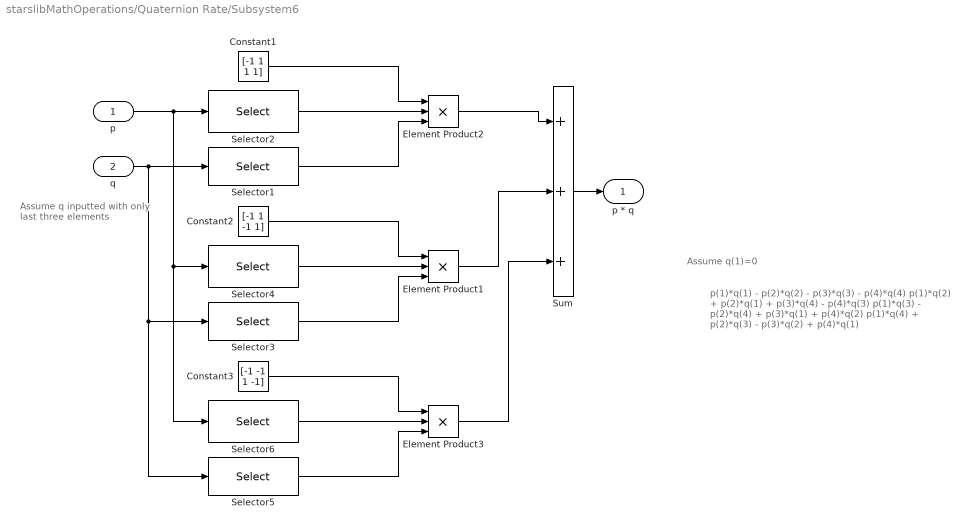
== system starslibMathOperations/Quaternion Rate/Subsystem6 ==
  note: p(1)*q(1) - p(2)*q(2) - p(3)*q(3) - p(4)*q(4)
      |
      | p(1)*q(2) + p(2)*q(1) + p(3)*q(4) - p(4)*q(3)
      |
      | p(1)*q(3) - p(2)*q(4) + p(3)*q(1) + p(4)*q(2)
      |
      | p(1)*q(4) + p(2)*q(3) - p(3)*q(2) + p(4)*q(1)
  note: Assume q(1)=0
  note: Assume q
      | inputted with only
      | last three elements
  p : Inport
  q : Inport  Port=2
  Constant1 : Constant  Value=[-1 1 1 1]
  Constant2 : Constant  Value=[-1 1 -1 1]
  Constant3 : Constant  Value=[-1 -1 1 -1]
  Element Product1 : Product  Inputs=3  RndMeth=Zero
  Element Product2 : Product  Inputs=3  RndMeth=Zero
  Element Product3 : Product  Inputs=3  RndMeth=Zero
  Selector1 : Selector  InputPortWidth=3  IndexOptions=Index vector (dialog)  Indices=[1 1 2 3]  OutputSizes=1
  Selector2 : Selector  InputPortWidth=4  IndexOptions=Index vector (dialog)  Indices=[2 1 1 1]  OutputSizes=1
  Selector3 : Selector  InputPortWidth=3  IndexOptions=Index vector (dialog)  Indices=[2 3 3 2]  OutputSizes=1
  Selector4 : Selector  InputPortWidth=4  IndexOptions=Index vector (dialog)  Indices=[3 3 2 2]  OutputSizes=1
  Selector5 : Selector  InputPortWidth=3  IndexOptions=Index vector (dialog)  Indices=[3 2 1 1]  OutputSizes=1
  Selector6 : Selector  InputPortWidth=4  IndexOptions=Index vector (dialog)  Indices=[4 4 4 3]  OutputSizes=1
  Sum : Sum  Inputs=+++
  p * q : Outport
  wires:
  Selector4/1 -> Element Product1/2
  Selector6/1 -> Element Product3/2
  Selector1/1 -> Element Product2/3
  Selector3/1 -> Element Product1/3
  Selector5/1 -> Element Product3/3
  Element Product2/1 -> Sum/1
  Element Product1/1 -> Sum/2
  Element Product3/1 -> Sum/3
  p/1 -> Selector2/1, Selector4/1, Selector6/1
  q/1 -> Selector1/1, Selector3/1, Selector5/1
  Sum/1 -> p * q/1
  Selector2/1 -> Element Product2/2
  Constant1/1 -> Element Product2/1
  Constant2/1 -> Element Product1/1
  Constant3/1 -> Element Product3/1

== system starslibMathOperations/nNormalize Vector/Divide by Zero Protection ==
  note: Replace magnitudes equal to 0 by 1
  M : Inport
  Constant : Constant
  Switch : Switch  Criteria=u2 ~= 0  ZeroCross=off  SaturateOnIntegerOverflow=off  InputSameDT=off
  M* : Outport
  wires:
  Switch/1 -> M*/1
  Constant/1 -> Switch/3
  M/1 -> Switch/2, Switch/1

== system starslibMathOperations/nNormalize Vector/Repeat Diminsion ==
  note: See initialization pane of mask for definition of A and B.
  M* : Inport
  Constant : Constant  Value=A  VectorParams1D=off
  Constant1 : Constant  Value=B  VectorParams1D=off
  Product : Product  Inputs=3  Multiplication=Matrix(*)  RndMeth=Zero
  Rep M* : Outport
  wires:
  Constant1/1 -> Product/3
  M*/1 -> Product/2
  Constant/1 -> Product/1
  Product/1 -> Rep M*/1

== system starslibMathOperations/nQuaternion Propagation/Orthonormality Error ==
  note: Zipfel, P. H., Modeling and Simulation of Aerospace Vehicle Dynamics, 2nd Ed., p372
  note: Quaternion orthonormality error.
  q : Inport  PortDimensions=[4,n]
  Constant : Constant
  Math Function : Math  Operator=square  SignedPower=on
  Sum of Elements : Sum  Inputs=+  CollapseMode=Specified dimension
  Sum1 : Sum  Inputs=|+-
  lambda : Outport  PortDimensions=[1,n]
  wires:
  Constant/1 -> Sum1/1
  Math Function/1 -> Sum of Elements/1
  Sum of Elements/1 -> Sum1/2
  q/1 -> Math Function/1
  Sum1/1 -> lambda/1
